simulink model "simu2016a"  (R2019a)
settings: Solver=FixedStepDiscrete  StartTime=0.0  StopTime=10  FixedStep=0.004  RelTol=1e-3
undefined symbols (not defined in the file): LF, serial
libraries: instrumentlib x2, dspfdesign x1
settings Model: Creator=14408  LastModifiedBy=Fahaxiki
settings OptimizationCC: DefaultParameterBehavior=Inlined  UseDivisionForNetSlopeComputation=on  UseFloatMulNetSlope=on  InlineInvariantSignals=on  PassReuseOutputArgsAs=Individual arguments  ZeroExternalMemoryAtStartup=off  ZeroInternalMemoryAtStartup=off  NoFixptDivByZeroProtection=on  EfficientFloat2IntCast=on  LifeSpan=1
settings DebuggingCC: ParameterTunabilityLossMsg=error  ArithmeticOperatorsInVariantConditions=warning
settings HardwareCC: ProdBitPerPointer=32  ProdBitPerSizeT=32  ProdBitPerPtrDiffT=32  ProdLargestAtomicInteger=Long  ProdLargestAtomicFloat=Double  ProdWordSize=32  ProdLongLongMode=on  ProdHWDeviceType=ARM Compatible->ARM Cortex
settings SFSimCC: MATLABDynamicMemAlloc=off
settings RTWCC: SystemTargetFile=ert.tlc  TemplateMakefile=ert_default_tmf
settings CodeAppCC: ForceParamTrailComments=on  IgnoreCustomStorageClasses=off  OperatorAnnotations=on  SimulinkDataObjDesc=on  SFDataObjDesc=on  CustomSymbolStrGlobalVar=rt$N$M  CustomSymbolStrType=$N$M  CustomSymbolStrFcn=$N$M$F  CustomSymbolStrMacro=$N$M  InsertBlockDesc=on  StateflowObjectComments=on
settings ERTTargetCC: TargetLangStandard=C99 (ISO)  GenerateSampleERTMain=on  IncludeMdlTerminateFcn=off  CombineSignalStateStructs=on  SupportAbsoluteTime=off  PurelyIntegerCode=on  SupportNonFinite=off  SupportComplex=off  InlinedParameterPlacement=NonHierarchical  ERTCustomFileTemplate=example_file_process.tlc  ERTFilePackagingFormat=CompactWithDataFile  MemSecPackage=Simulink

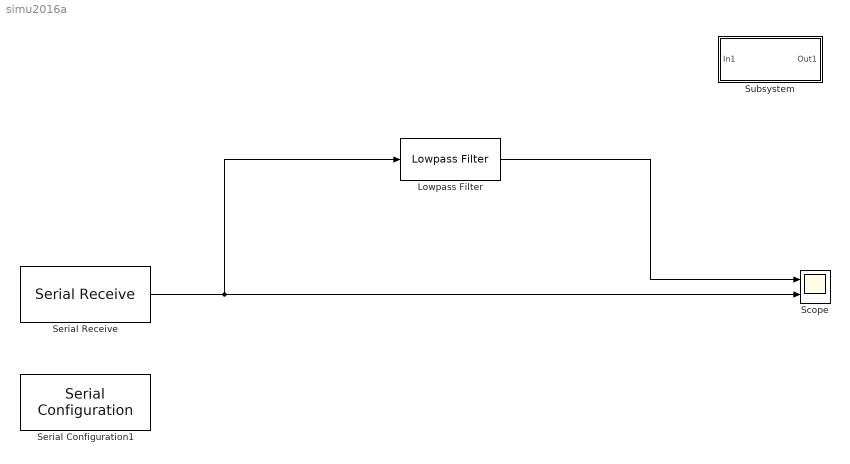
== system simu2016a ==
  Lowpass Filter : dspfdesign/Lowpass Filter  FilterType=FIR  DesignForMinimumOrder=on  FilterOrder=50  PassbandFrequency=1  StopbandFrequency=49  PassbandRipple=0.1  StopbandAttenuation=80  InheritSampleRate=off  SampleRate=500  SimulateUsing=Interpreted execution  roundingMode=Floor  coeffsDataTypeStr=fixdt(1,16)
  Scope : Scope  NumInputPorts=2
  Serial Configuration1 : instrumentlib/Serial Configuration  Priority=-200000  ComPortMenu=<Please select a port...>  ComPort=COM11  ObjConstructor=serial('COM11');  BaudRate=115200  DataBits=8  Parity=none  StopBits=1  FlowControl=none  Timeout=10  ByteOrder=LittleEndian
  Serial Receive : instrumentlib/Serial Receive  ComPortMenu=<Please select a port...>  ComPort=COM11  ObjConstructor=serial('COM11');  Terminator=LF ('\n')  DataSize=[1 1]  DataType=uint32  EnableBlockingMode=on  ActionDataUnavailable=Output last received value  CustomValue=0  SampleTime=0.004
  Subsystem : Subsystem
  wires:
  Serial Receive/1 -> Lowpass Filter/1, Scope/2
  Lowpass Filter/1 -> Scope/1

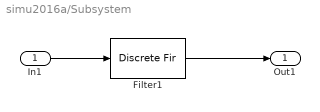
== system simu2016a/Subsystem ==
  In1 : Inport
  Filter1 : DiscreteFir  Tag=BlockMethodSubSystem  Coefficients=[0.000613080072987561963 0.00121339762389561351 0.00230145427824709125 0.00389947763361839315 0.00609180850498943025 0.00893213654541564865 0.012429813845641173 0.0165404369774478366 0.0211589370264876862 0.026121422966647885 0.0312111824196520914 0.0361734681521403215 0.0407339974469950114 0.0446227413022574487 0.0475966424855195983 0.0494633136629805126 0.0500999783903156373 0.0494633136629805126 0.0475966424855195983 0.0446227413022574487 0.0407339974469950114 0.0361734681521403215 0.0312111824196520914 0.026121422966647885 0.0211589370264876862 0.0165404369774478366 0.012429813845641173 0.00893213654541564865 0.00609180850498943025 0.00389947763361839315 0.00230145427824709125 0.00121339762389561351 0.000613080072987561963]  InputProcessing=Columns as channels (frame based)
  Out1 : Outport
  wires:
  In1/1 -> Filter1/1
  Filter1/1 -> Out1/1
